simulink subsystem "Global_fault_injection"  (R2025a)
settings: Solver=VariableStepAuto  StartTime=0.0  StopTime=10.0  RelTol=1e-3
settings Model: Creator=gurt1  LastModifiedBy=gurt1

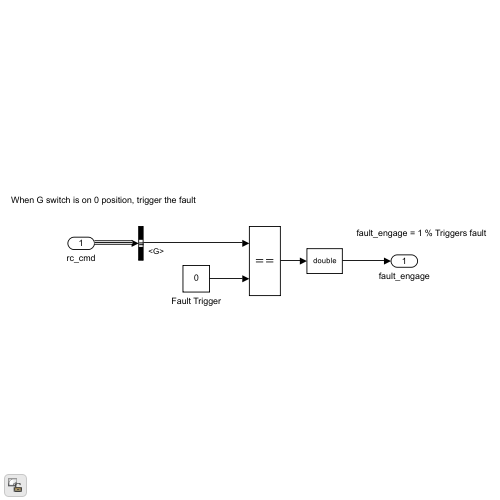
[thumbnail: Simulink's stored preview of the top-level diagram]
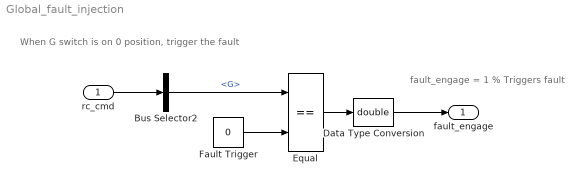
== system Global_fault_injection ==
  note: fault_engage = 1 % Triggers fault
  note: When G switch is on 0 position, trigger the fault
  rc_cmd : Inport
  Bus Selector2 : BusSelector  OutputSignals=switches.G
  Data Type Conversion : DataTypeConversion  OutDataTypeStr=double  SaturateOnIntegerOverflow=off  RndMeth=Floor
  Equal : RelationalOperator  Operator===  OutDataTypeStr=boolean  RndMeth=Simplest  InputSameDT=off
  Fault Trigger : Constant  Value=0  OutDataTypeStr=Inherit: Inherit via back propagation
  fault_engage : Outport
  wires:
  Bus Selector2/1 -> Equal/1  "<G>"
  rc_cmd/1 -> Bus Selector2/1
  Fault Trigger/1 -> Equal/2
  Equal/1 -> Data Type Conversion/1
  Data Type Conversion/1 -> fault_engage/1
